simulink subsystem "coolantTemp"  (R2022b)
settings: Solver=VariableStepAuto  StartTime=0.0  StopTime=10.0  RelTol=1e-3
libraries: coolant x2
settings Model: Creator=serga  LastModifiedBy=serga

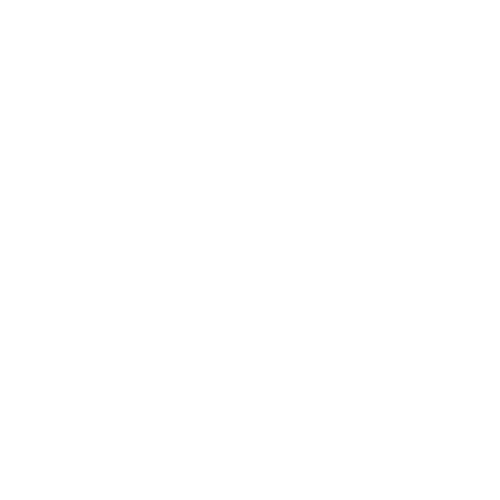
[thumbnail: Simulink's stored preview of the top-level diagram]
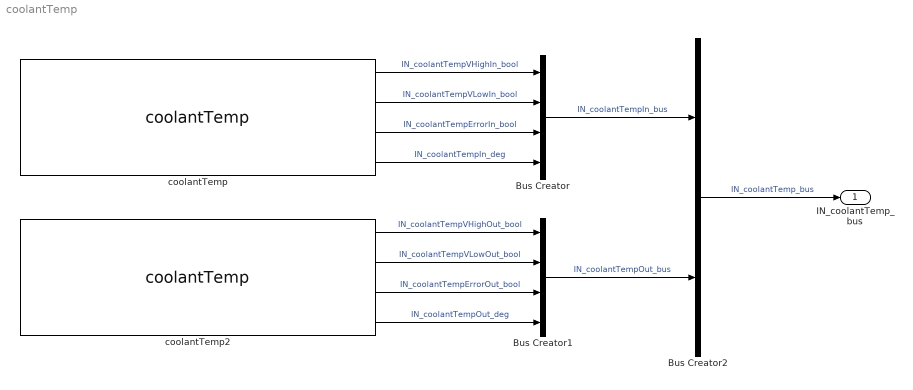
== system coolantTemp ==
  Bus Creator : BusCreator  Inputs=4
  Bus Creator1 : BusCreator  Inputs=4
  Bus Creator2 : BusCreator  Inputs=2
  coolantTemp : coolant/coolantTemp  pos='In'
  coolantTemp2 : coolant/coolantTemp  pos='Out'
  IN_coolantTemp_bus : Outport
  wires:
  Bus Creator2/1 -> IN_coolantTemp_bus/1  "IN_coolantTemp_bus"
  Bus Creator/1 -> Bus Creator2/1  "IN_coolantTempIn_bus"
  Bus Creator1/1 -> Bus Creator2/2  "IN_coolantTempOut_bus"
  coolantTemp2/4 -> Bus Creator1/4  "IN_coolantTempOut_deg"
  coolantTemp2/3 -> Bus Creator1/3  "IN_coolantTempErrorOut_bool"
  coolantTemp2/2 -> Bus Creator1/2  "IN_coolantTempVLowOut_bool"
  coolantTemp2/1 -> Bus Creator1/1  "IN_coolantTempVHighOut_bool"
  coolantTemp/4 -> Bus Creator/4  "IN_coolantTempIn_deg"
  coolantTemp/3 -> Bus Creator/3  "IN_coolantTempErrorIn_bool"
  coolantTemp/2 -> Bus Creator/2  "IN_coolantTempVLowIn_bool"
  coolantTemp/1 -> Bus Creator/1  "IN_coolantTempVHighIn_bool"
